simulink subsystem "directFFcontroller"  (R2021a)
settings: Solver=VariableStepAuto  StartTime=0.0  StopTime=10.0  RelTol=1e-3
settings Model: Creator=chukh  LastModifiedBy=brandon

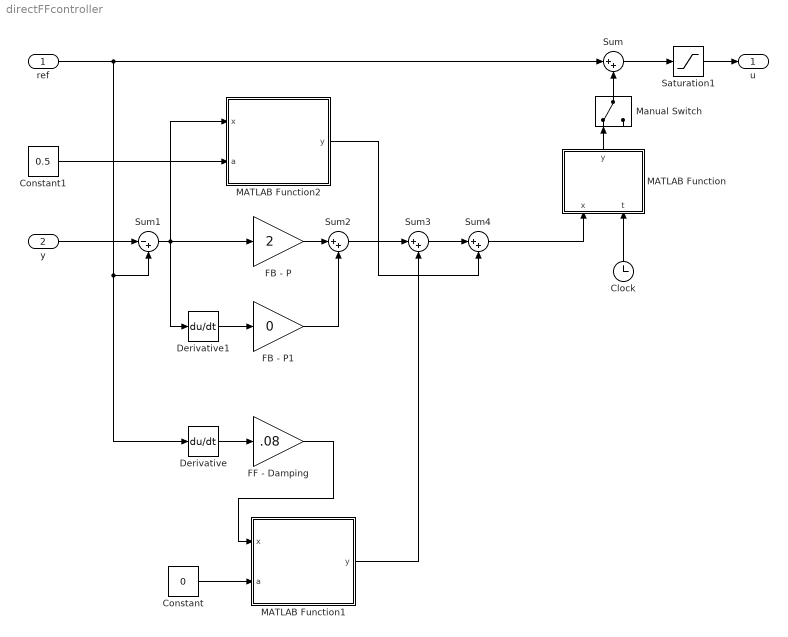
== system directFFcontroller ==
  ref : Inport
  y : Inport  Port=2
  Clock : Clock
  Constant : Constant  Value=0
  Constant1 : Constant  Value=0.5
  Derivative : Derivative
  Derivative1 : Derivative
  FB - P : Gain  Gain=2
  FB - P1 : Gain  Gain=0
  FF - Damping : Gain  Gain=.08
  MATLAB Function : MATLAB Function  TreatAsAtomicUnit=on
  MATLAB Function1 : MATLAB Function  TreatAsAtomicUnit=on
  MATLAB Function2 : MATLAB Function  TreatAsAtomicUnit=on
  Manual Switch : ManualSwitch
  Saturation1 : Saturate  UpperLimit=1  LowerLimit=0
  Sum{,2..4} (4 alike) : Sum  Inputs=|++
  Sum1 : Sum  Inputs=|-+
  u : Outport
  wires:
  Saturation1/1 -> u/1
  ref/1 -> Sum/1, Derivative/1, Sum1/2
  FB - P/1 -> Sum2/1
  Manual Switch/1 -> Sum/2
  y/1 -> Sum1/1
  Derivative/1 -> FF - Damping/1
  Sum1/1 -> FB - P/1, Derivative1/1, MATLAB Function2/1(x)
  FB - P1/1 -> Sum2/2
  Derivative1/1 -> FB - P1/1
  Clock/1 -> MATLAB Function/2(t)
  MATLAB Function/1(y) -> Manual Switch/1
  Sum/1 -> Saturation1/1
  MATLAB Function1/1(y) -> Sum3/2
  Constant/1 -> MATLAB Function1/2(a)
  Sum2/1 -> Sum3/1
  FF - Damping/1 -> MATLAB Function1/1(x)
  Sum3/1 -> Sum4/1
  Sum4/1 -> MATLAB Function/1(x)
  Constant1/1 -> MATLAB Function2/2(a)
  MATLAB Function2/1(y) -> Sum4/2

== matlab function directFFcontroller/MATLAB Function1 ==
  data: x input; a input; y output
function y = deadzoneInverse(x,a)
y = x+a*sign(x);
end

== matlab function directFFcontroller/MATLAB Function2 ==
  data: x input; a input; y output
function y = deadzoneInverse(x,a)

if abs(x) <= 0.03
  y = a*sign(x)*x;
else
  y = 0;  
end

end

== matlab function directFFcontroller/MATLAB Function ==
  data: x input; t input; y output
function y = smoothstep(x,t)
y = x*min(0.2*t,1);
end
